simulink model "diagramme_fonctionnel"  (R2023a)
settings: Solver=ode45  StartTime=0.0  StopTime=150  RelTol=1e-7  EnableMultiTasking=on
settings Model: Creator=LiberT  LastModifiedBy=spbou6
settings SolverCC: AlgebraicLoopSolver=TrustRegion
settings DataIOCC: LimitDataPoints=on  SaveFormat=Array  SignalLoggingSaveFormat=ModelDataLogs  ReturnWorkspaceOutputs=off
settings OptimizationCC: BlockReduction=off  BooleanDataType=off  ExpressionDepthLimit=2147483647  InitFltsAndDblsToZero=on  LifeSpan=inf
settings DebuggingCC: SaveWithParameterizedLinksMsg=none  UnderspecifiedInitializationDetection=Classic  MergeDetectMultiDrivingBlocksExec=none  SignalResolutionControl=TryResolveAllWithWarning  MultiTaskDSMMsg=warning  MultiTaskCondExecSysMsg=none  FcnCallInpInsideContextMsg=warning  UnconnectedInputMsg=warning  UnconnectedOutputMsg=warning  UnconnectedLineMsg=warning  StateNameClashWarn=warning  SFUnexpectedBacktrackingDiag=warning  SFNoUnconditionalDefaultTransitionDiag=warning  SFExecutionAtInitializationDiag=none  ArithmeticOperatorsInVariantConditions=warning
settings HardwareCC: ProdBitPerPointer=32  ProdBitPerSizeT=32  ProdBitPerPtrDiffT=32  ProdLargestAtomicFloat=None  ProdIntDivRoundTo=Undefined  ProdEndianess=Unspecified  ProdWordSize=32  ProdHWDeviceType=32-bit Generic  TargetUnknown=on
settings ModelReferenceCC: EnableRefExpFcnMdlSchedulingChecks=on  PropagateSignalLabelsOutOfModel=off
settings SFSimCC: SimUseLocalCustomCode=off  CustomCodeUndefinedFunction=UseInterfaceOnly
settings RTWCC: RTWUseLocalCustomCode=off
settings CodeAppCC: StateflowObjectComments=on
settings GRTTargetCC: TargetFcnLib=ansi_tfl_tmw.mat  TargetLangStandard=C89/C90 (ANSI)  ModelReferenceCompliant=off  CompOptLevelCompliant=off  CombineOutputUpdateFcns=off  MatFileLogging=off  GRTInterface=on
settings ConfigComp: CovMetricSettings=dw  CovSaveCumulativeToWorkspaceVar=on  CovSaveSingleToWorkspaceVar=on  CovExternalEMLEnable=off

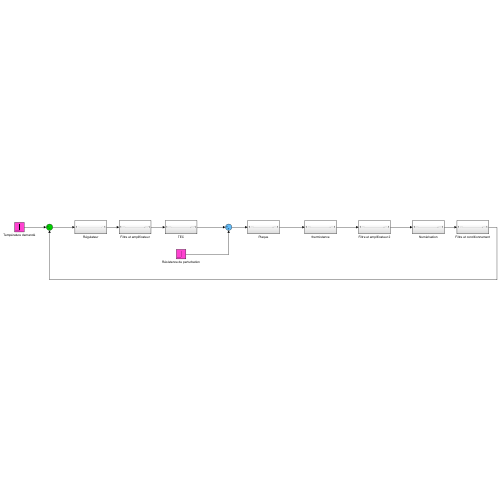
[thumbnail: Simulink's stored preview of the top-level diagram]
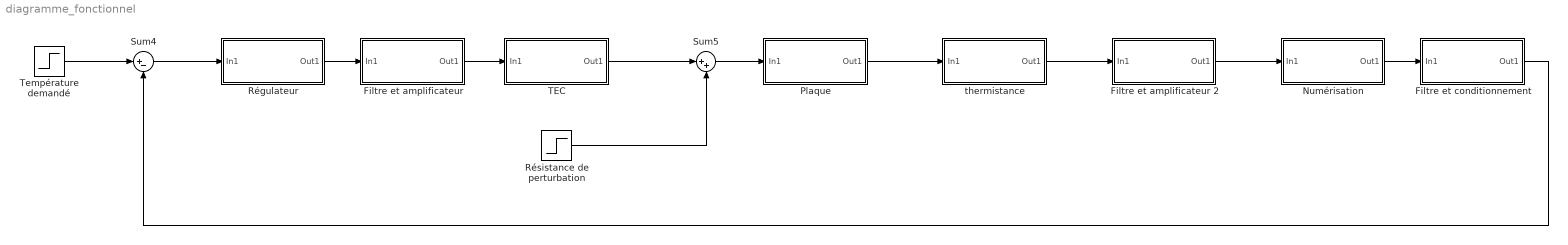
== system diagramme_fonctionnel ==
  Filtre et amplificateur : Subsystem
  Filtre et amplificateur 2 : Subsystem
  Filtre et conditionnement : Subsystem
  Numérisation : Subsystem
  Plaque : Subsystem
  Régulateur : Subsystem
  Résistance de perturbation : Step  SampleTime=0
  Sum4 : Sum  Inputs=|+-  InputSameDT=on  SaturateOnIntegerOverflow=on  OutDataTypeStr=Inherit: Same as first input
  Sum5 : Sum  Inputs=|++  InputSameDT=on  SaturateOnIntegerOverflow=on  OutDataTypeStr=Inherit: Same as first input
  TEC : Subsystem
  Température demandé : Step  SampleTime=0
  thermistance : Subsystem
  wires:
  Filtre et conditionnement/1(Out1) -> Sum4/2
  Sum4/1 -> Régulateur/1(In1)
  Température demandé/1 -> Sum4/1
  Régulateur/1(Out1) -> Filtre et amplificateur/1(In1)
  Filtre et amplificateur/1(Out1) -> TEC/1(In1)
  Résistance de perturbation/1 -> Sum5/2
  TEC/1(Out1) -> Sum5/1
  Sum5/1 -> Plaque/1(In1)
  Plaque/1(Out1) -> thermistance/1(In1)
  thermistance/1(Out1) -> Filtre et amplificateur 2/1(In1)
  Filtre et amplificateur 2/1(Out1) -> Numérisation/1(In1)
  Numérisation/1(Out1) -> Filtre et conditionnement/1(In1)

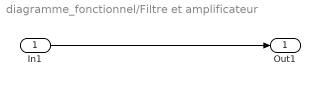
== system diagramme_fonctionnel/Filtre et amplificateur ==
  In1 : Inport
  Out1 : Outport
  wires:
  In1/1 -> Out1/1

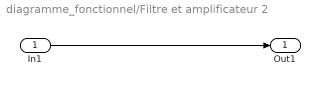
== system diagramme_fonctionnel/Filtre et amplificateur 2 ==
  In1 : Inport
  Out1 : Outport
  wires:
  In1/1 -> Out1/1

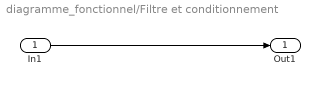
== system diagramme_fonctionnel/Filtre et conditionnement ==
  In1 : Inport
  Out1 : Outport
  wires:
  In1/1 -> Out1/1

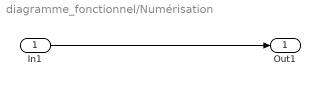
== system diagramme_fonctionnel/Numérisation ==
  In1 : Inport
  Out1 : Outport
  wires:
  In1/1 -> Out1/1

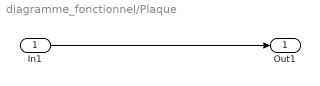
== system diagramme_fonctionnel/Plaque ==
  In1 : Inport
  Out1 : Outport
  wires:
  In1/1 -> Out1/1

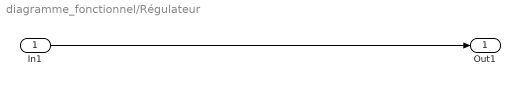
== system diagramme_fonctionnel/Régulateur ==
  In1 : Inport
  Out1 : Outport
  wires:
  In1/1 -> Out1/1

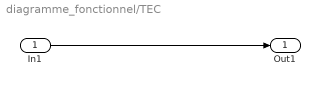
== system diagramme_fonctionnel/TEC ==
  In1 : Inport
  Out1 : Outport
  wires:
  In1/1 -> Out1/1

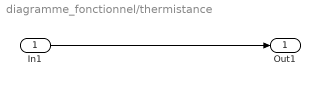
== system diagramme_fonctionnel/thermistance ==
  In1 : Inport
  Out1 : Outport
  wires:
  In1/1 -> Out1/1
